simulink model "URM_IOKU_3b"  (R2014a)
settings: Solver=ode45  StartTime=0.0  StopTime=18  RelTol=1e-3
values from neighbouring files (symbols this model uses):
  a1 = 2    [URM_SP.m]
  a2 = 1.5    [URM_SP.m]
  a3 = 0.5    [URM_SP.m]
  D = linspace(d1,d2,n)    [URM_SP.m]
libraries: mblibv1 x12, simulink x3
settings Model: Creator=kajak_000  LastModifiedBy=kajak_000
settings SimMechanicsCC: VisDuringSimulation=on

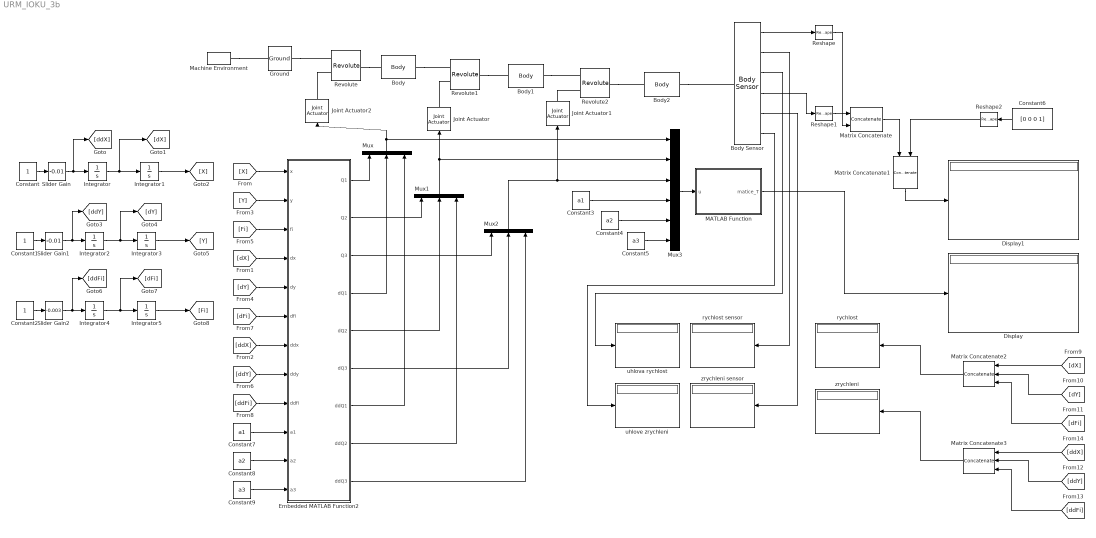
== system URM_IOKU_3b ==
  Body : mblibv1/Bodies/Body  LConnTagsString=CS1  RConnTagsString=CS2  UpdateFromCAD=off  DialogClass=MechanicalBodyBlock  Mass=1  MassUnits=kg  InertiaUnits=kg*m^2  Inertia=eye(3)  Shape=Cylinder  ShapeDims=[1 1]  ShapeUnits=m  ShapeUse=false  Density=1  DensityUnits=kg/m^3  DensityUse=false  GraphicsMode=MACHINE_DEFAULT  BodyColorSelMode=MACHINE_DEFAULT  BodyColor=[1 0 0]  AttachedToCS=CG  CG=Left$CG$rameno1.CG$WORLD$WORLD$m$[0 0 0]$Euler X-Y-Z$deg$WORLD$false$none  WorkingFrames=Left$CS1$rameno1.A$World$World$m$[0 0 0]$Euler X-Y-Z$deg$WORLD$true$none#Right$CS2$rameno1.B$World$World$m$[0 0 0]$Euler X-Y-Z$deg$WORLD$true$none  CGPos=rameno1.CG  CGRot=[0 0 0]  CS0Pos=[]  CS0Rot=[]  CS1Pos=rameno1.A  CS1Rot=[0 0 0]  CS2Pos=rameno1.B  CS2Rot=[0 0 0]  CS3Pos=[]  CS3Rot=[]  CS4Pos=[]  CS4Rot=[]  CS5Pos=[]  CS5Rot=[]  CS6Pos=[]  CS6Rot=[]  CS7Pos=[]  CS7Rot=[]  CS8Pos=[]  CS8Rot=[]  CS9Pos=[]  CS9Rot=[]  CS10Pos=[]  CS10Rot=[]  CS11Pos=[]  CS11Rot=[]  CS12Pos=[]  CS12Rot=[]  CS13Pos=[]  CS13Rot=[]  CS14Pos=[]  CS14Rot=[]  CS15Pos=[]  CS15Rot=[]  CS16Pos=[]  CS16Rot=[]  CS17Pos=[]  CS17Rot=[]  CS18Pos=[]  CS18Rot=[]  CS19Pos=[]  CS19Rot=[]  CS20Pos=[]  CS20Rot=[]
  Body Sensor : mblibv1/Sensors &  Actuators/Body Sensor  UpdateFromCAD=off  PhysicalDomain=Mechanical  PortType=blob  Muxed=off  Pose=on  Angle=on  AngleUnits=deg  ArcVelocity=on  ArcVelocityUnits=rad/s  ArcAcceleration=on  ArcAccelerationUnits=rad/s^2  CoordPosition=on  CoordPositionUnits=m  Velocity=on  VelocityUnits=m/s  Acceleration=on  AccelerationUnits=m/s^2  Quaternion=on  QuaternionDT=off  QuaternionDDT=off  QuaternionUnits=off  OutputVector="[ 3  3  3  9  3  3]"  ActiveIO=on  Width=24  DialogClass=MechanicalSensorBlock  ReferenceFrame=Absolute (World)
  Body1 : mblibv1/Bodies/Body  LConnTagsString=CS1  RConnTagsString=CS2  UpdateFromCAD=off  DialogClass=MechanicalBodyBlock  Mass=1  MassUnits=kg  InertiaUnits=kg*m^2  Inertia=eye(3)  Shape=Cylinder  ShapeDims=[1 1]  ShapeUnits=m  ShapeUse=false  Density=1  DensityUnits=kg/m^3  DensityUse=false  GraphicsMode=MACHINE_DEFAULT  BodyColorSelMode=MACHINE_DEFAULT  BodyColor=[1 0 0]  AttachedToCS=CG  CG=Left$CG$rameno2.CG$WORLD$WORLD$m$[0 0 0]$Euler X-Y-Z$deg$WORLD$false$none  WorkingFrames=Left$CS1$rameno2.A$World$World$m$[0 0 0]$Euler X-Y-Z$deg$WORLD$true$none#Right$CS2$rameno2.B$World$World$m$[0 0 0]$Euler X-Y-Z$deg$WORLD$true$none  CGPos=rameno2.CG  CGRot=[0 0 0]  CS0Pos=[]  CS0Rot=[]  CS1Pos=rameno2.A  CS1Rot=[0 0 0]  CS2Pos=rameno2.B  CS2Rot=[0 0 0]  CS3Pos=[]  CS3Rot=[]  CS4Pos=[]  CS4Rot=[]  CS5Pos=[]  CS5Rot=[]  CS6Pos=[]  CS6Rot=[]  CS7Pos=[]  CS7Rot=[]  CS8Pos=[]  CS8Rot=[]  CS9Pos=[]  CS9Rot=[]  CS10Pos=[]  CS10Rot=[]  CS11Pos=[]  CS11Rot=[]  CS12Pos=[]  CS12Rot=[]  CS13Pos=[]  CS13Rot=[]  CS14Pos=[]  CS14Rot=[]  CS15Pos=[]  CS15Rot=[]  CS16Pos=[]  CS16Rot=[]  CS17Pos=[]  CS17Rot=[]  CS18Pos=[]  CS18Rot=[]  CS19Pos=[]  CS19Rot=[]  CS20Pos=[]  CS20Rot=[]
  Body2 : mblibv1/Bodies/Body  LConnTagsString=CS1  RConnTagsString=CS2  UpdateFromCAD=off  DialogClass=MechanicalBodyBlock  Mass=1  MassUnits=kg  InertiaUnits=kg*m^2  Inertia=eye(3)  Shape=Cylinder  ShapeDims=[1 1]  ShapeUnits=m  ShapeUse=false  Density=1  DensityUnits=kg/m^3  DensityUse=false  GraphicsMode=MACHINE_DEFAULT  BodyColorSelMode=MACHINE_DEFAULT  BodyColor=[1 0 0]  AttachedToCS=CG  CG=Left$CG$rameno3.CG$WORLD$WORLD$m$[0 0 0]$Euler X-Y-Z$deg$WORLD$false$none  WorkingFrames=Left$CS1$rameno3.A$World$World$m$[0 0 0]$Euler X-Y-Z$deg$WORLD$true$none#Right$CS2$rameno3.B$World$World$m$[0 0 0]$Euler X-Y-Z$deg$WORLD$true$none  CGPos=rameno3.CG  CGRot=[0 0 0]  CS0Pos=[]  CS0Rot=[]  CS1Pos=rameno3.A  CS1Rot=[0 0 0]  CS2Pos=rameno3.B  CS2Rot=[0 0 0]  CS3Pos=[]  CS3Rot=[]  CS4Pos=[]  CS4Rot=[]  CS5Pos=[]  CS5Rot=[]  CS6Pos=[]  CS6Rot=[]  CS7Pos=[]  CS7Rot=[]  CS8Pos=[]  CS8Rot=[]  CS9Pos=[]  CS9Rot=[]  CS10Pos=[]  CS10Rot=[]  CS11Pos=[]  CS11Rot=[]  CS12Pos=[]  CS12Rot=[]  CS13Pos=[]  CS13Rot=[]  CS14Pos=[]  CS14Rot=[]  CS15Pos=[]  CS15Rot=[]  CS16Pos=[]  CS16Rot=[]  CS17Pos=[]  CS17Rot=[]  CS18Pos=[]  CS18Rot=[]  CS19Pos=[]  CS19Rot=[]  CS20Pos=[]  CS20Rot=[]
  Constant : Constant
  Constant1 : Constant
  Constant2 : Constant
  Constant3 : Constant  Value=a1
  Constant4 : Constant  Value=a2
  Constant5 : Constant  Value=a3
  Constant6 : Constant  Value=[0 0 0 1]
  Constant7 : Constant  Value=a1
  Constant8 : Constant  Value=a2
  Constant9 : Constant  Value=a3
  Display : Display
  Display1 : Display
  Embedded MATLAB Function2 : MATLAB Function  TreatAsAtomicUnit=on
  Ground : mblibv1/Bodies/Ground  UpdateFromCAD=off  LeftPortType=env  RightPortType=workingframe  PhysicalDomain=Mechanical  DialogClass=GroundBlock  CoordPosition=rameno1.A  CoordPositionUnits=m  StateVectorMgrId=7  MachineId=[8 0]  ShowEnvPort=on  ParameterChecksum=[1572609533, 1849027617, 4062556937, 1555680548]  TopologyChecksum=[1622869580, 615649969, 3102652873, 2552126148]
  Integrator{,1..5} (6 alike) : Integrator
  Joint Actuator : mblibv1/Sensors &  Actuators/Joint Actuator  UpdateFromCAD=off  PhysicalDomain=Mechanical  PortType=blob  ActuationStyle=Motion  AngleUnits=rad  ArcVelocityUnits=rad/s  ArcAccelerationUnits=rad/s^2  CoordPositionUnits=m  VelocityUnits=m/s  AccelerationUnits=m/s^2  ForceUnits=N  TorqueUnits=N*m  ActiveIO=on  Width=3  DialogClass=MechanicalActuatorBlock  Primitive=R1  ReferenceFrame=Absolute (World)
  Joint Actuator1 : mblibv1/Sensors &  Actuators/Joint Actuator  UpdateFromCAD=off  PhysicalDomain=Mechanical  PortType=blob  ActuationStyle=Motion  AngleUnits=rad  ArcVelocityUnits=rad/s  ArcAccelerationUnits=rad/s^2  CoordPositionUnits=m  VelocityUnits=m/s  AccelerationUnits=m/s^2  ForceUnits=N  TorqueUnits=N*m  ActiveIO=on  Width=3  DialogClass=MechanicalActuatorBlock  Primitive=R1  ReferenceFrame=Absolute (World)
  Joint Actuator2 : mblibv1/Sensors &  Actuators/Joint Actuator  UpdateFromCAD=off  PhysicalDomain=Mechanical  PortType=blob  ActuationStyle=Motion  AngleUnits=rad  ArcVelocityUnits=rad/s  ArcAccelerationUnits=rad/s^2  CoordPositionUnits=m  VelocityUnits=m/s  AccelerationUnits=m/s^2  ForceUnits=N  TorqueUnits=N*m  ActiveIO=on  Width=3  DialogClass=MechanicalActuatorBlock  Primitive=R1  ReferenceFrame=Absolute (World)
  MATLAB Function : MATLAB Function  TreatAsAtomicUnit=on
  Machine Environment : mblibv1/Bodies/Machine Environment  PortType=env  PhysicalDomain=Mechanical  DialogTemplateClass=MECH.MachineEnvironment  SyncWhenCopied=off  Gravity=[0 0 0]  GravityUnits=m/s^2  GravityAsSignal=off  Dimensionality=Auto-detect  AnalysisType=Forward dynamics  LinearAssemblyTolerance=1e-3  LinearAssemblyToleranceUnits=m  AngularAssemblyTolerance=1e-3  AngularAssemblyToleranceUnits=rad  ConstraintSolverType=Stabilizing  ConstraintRelTolerance=1e-4  ConstraintAbsTolerance=1e-4  UseRobustSingularityHandling=off  RedundancyAnalysisToleranceType=Automatically select tolerance  RedundancyAnalysisTolerance=1e-14  StatePerturbationType=Fixed  PerturbationSize=1e-5  VisualizeMachine=on  BodyVisualizationType=Use model default body geometries  BodyColorSelMode=Use model default  DefaultBodyColor=[1 0 0]
  Matrix Concatenate : Concatenate  Mode=Multidimensional array  ConcatenateDimension=2
  Matrix Concatenate1 : Concatenate  Mode=Multidimensional array
  Matrix Concatenate2 : Concatenate  NumInputs=3  ConcatenateDimension=2
  Matrix Concatenate3 : Concatenate  NumInputs=3  ConcatenateDimension=2
  Mux : Mux  Inputs=3
  Mux1 : Mux  Inputs=3
  Mux2 : Mux  Inputs=3
  Mux3 : Mux  Inputs=6
  Reshape : Reshape  OutputDimensionality=Column vector (2-D)
  Reshape1 : Reshape  OutputDimensionality=Customize  OutputDimensions=[3,3]
  Reshape2 : Reshape  OutputDimensionality=Row vector (2-D)  OutputDimensions=[3,1]
  Revolute : mblibv1/Joints/Revolute  LConnTagsString=__newl0|SA1  RConnTagsString=__newr0  UpdateFromCAD=off  NumSAPorts=1  CutJoint=off  MarkAsCut=off  Primitives=prismatic  PrimitiveProps=R1$World$rameno1.osa$revolute  DialogClass=JointBlock  R1Axis=rameno1.osa
  Revolute1 : mblibv1/Joints/Revolute  LConnTagsString=__newl0|SA1  RConnTagsString=__newr0  UpdateFromCAD=off  NumSAPorts=1  CutJoint=off  MarkAsCut=off  Primitives=prismatic  PrimitiveProps=R1$World$rameno2.osa$revolute  DialogClass=JointBlock  R1Axis=rameno2.osa
  Revolute2 : mblibv1/Joints/Revolute  LConnTagsString=__newl0|SA1  RConnTagsString=__newr0  UpdateFromCAD=off  NumSAPorts=1  CutJoint=off  MarkAsCut=off  Primitives=prismatic  PrimitiveProps=R1$World$rameno3.osa$revolute  DialogClass=JointBlock  R1Axis=rameno3.osa
  Slider Gain : simulink/Math Operations/Slider Gain  low=-2  gain=-0.01  high=2
  Slider Gain1 : simulink/Math Operations/Slider Gain  low=-2  gain=-0.01  high=2
  Slider Gain2 : simulink/Math Operations/Slider Gain  low=-2  gain=-0.003  high=2
  rychlost : Display
  rychlost sensor : Display
  uhlova rychlost : Display
  uhlove zrychleni : Display
  zrychleni : Display
  zrychleni sensor : Display
  wires:
  Slider Gain/1 -> [ddX], Integrator/1
  Constant/1 -> Slider Gain/1
  Constant3/1 -> Mux3/4
  Constant4/1 -> Mux3/5
  Constant5/1 -> Mux3/6
  Mux3/1 -> MATLAB Function/1(u)
  MATLAB Function/1(matice_T) -> Display/1
  Body Sensor/1 -> Reshape/1
  Body Sensor/4 -> Reshape1/1
  Reshape1/1 -> Matrix Concatenate/1
  Reshape/1 -> Matrix Concatenate/2
  Constant6/1 -> Reshape2/1
  Matrix Concatenate/1 -> Matrix Concatenate1/1
  Reshape2/1 -> Matrix Concatenate1/2
  Matrix Concatenate1/1 -> Display1/1
  Integrator/1 -> [dX], Integrator1/1
  Slider Gain1/1 -> [ddY], Integrator2/1
  Constant1/1 -> Slider Gain1/1
  Integrator2/1 -> [dY], Integrator3/1
  Body Sensor/2 -> rychlost sensor/1
  Body Sensor/5 -> zrychleni sensor/1
  Body Sensor/3 -> uhlova rychlost/1
  Body Sensor/6 -> uhlove zrychleni/1
  [X] -> Embedded MATLAB Function2/1(x)
  Integrator1/1 -> [X]
  Integrator3/1 -> [Y]
  Slider Gain2/1 -> [ddFi], Integrator4/1
  Constant2/1 -> Slider Gain2/1
  Integrator4/1 -> [dFi], Integrator5/1
  Integrator5/1 -> [Fi]
  Mux/1 -> Joint Actuator2/1, Mux3/1
  Mux1/1 -> Joint Actuator/1, Mux3/2
  Mux2/1 -> Joint Actuator1/1, Mux3/3
  Matrix Concatenate2/1 -> rychlost/1
  [dX] -> Matrix Concatenate2/1
  [dY] -> Matrix Concatenate2/2
  [dFi] -> Matrix Concatenate2/3
  Matrix Concatenate3/1 -> zrychleni/1
  [ddX] -> Matrix Concatenate3/1
  [ddY] -> Matrix Concatenate3/2
  [ddFi] -> Matrix Concatenate3/3
  [Y] -> Embedded MATLAB Function2/2(y)
  [dX] -> Embedded MATLAB Function2/4(dx)
  [dY] -> Embedded MATLAB Function2/5(dy)
  [dFi] -> Embedded MATLAB Function2/6(dfi)
  [ddY] -> Embedded MATLAB Function2/8(ddy)
  [ddX] -> Embedded MATLAB Function2/7(ddx)
  [Fi] -> Embedded MATLAB Function2/3(fi)
  [ddFi] -> Embedded MATLAB Function2/9(ddfi)
  Constant7/1 -> Embedded MATLAB Function2/10(a1)
  Constant8/1 -> Embedded MATLAB Function2/11(a2)
  Constant9/1 -> Embedded MATLAB Function2/12(a3)
  Embedded MATLAB Function2/1(Q1) -> Mux/1
  Embedded MATLAB Function2/4(dQ1) -> Mux/2
  Embedded MATLAB Function2/7(ddQ1) -> Mux/3
  Embedded MATLAB Function2/2(Q2) -> Mux1/1
  Embedded MATLAB Function2/5(dQ2) -> Mux1/2
  Embedded MATLAB Function2/8(ddQ2) -> Mux1/3
  Embedded MATLAB Function2/3(Q3) -> Mux2/1
  Embedded MATLAB Function2/6(dQ3) -> Mux2/2
  Embedded MATLAB Function2/9(ddQ3) -> Mux2/3
  connections:
  Machine Environment/RConn1 -- Ground/LConn1
  Ground/RConn1 -- Revolute/LConn1
  Revolute/RConn1 -- Body/LConn1
  Body/RConn1 -- Revolute1/LConn1
  Revolute1/RConn1 -- Body1/LConn1
  Body1/RConn1 -- Revolute2/LConn1
  Revolute2/RConn1 -- Body2/LConn1
  Body2/RConn1 -- Body Sensor/LConn1
  Joint Actuator/RConn1 -- Revolute1/LConn2
  Joint Actuator1/RConn1 -- Revolute2/LConn2
  Joint Actuator2/RConn1 -- Revolute/LConn2

== matlab function URM_IOKU_3b/MATLAB Function ==
  data: u input; matice_T output
function matice_T = DGM_funkce(u)
Q1 = u(1); % poloha
Q2 = u(4);
Q3 = u(7);
a1 = u(10);
a2 = u(11);
a3 = u(12);
matice_T = zeros(4);

x = a3 * cos(Q1 + Q2 + Q3) + a2 * cos(Q1 + Q2) + a1 * cos(Q1);
y = a3 * sin(Q1 + Q2 + Q3) + a2 * sin(Q1 + Q2) + a1 * sin(Q1);
vysledny_uhel = Q1 + Q2 + Q3; 

matice_T = [ cos(vysledny_uhel),-sin(vysledny_uhel),0,x;
            sin(vysledny_uhel),cos(vysledny_uhel),0,y;
            0,0,1,0;
            0,0,0,1 ];
       
end

== matlab function URM_IOKU_3b/Embedded MATLAB Function2 ==
  data: Q1 output; Q2 output; Q3 output; dQ1 output; dQ2 output; dQ3 output; ddQ1 output; ddQ2 output; ddQ3 output; x input; y input; fi input; dx input; dy input; dfi input; ddx input; ddy input; ddfi input; a1 input; a2 input; a3 input
function [Q1, Q2, Q3, dQ1, dQ2, dQ3, ddQ1, ddQ2, ddQ3] = IOKU(x, y, fi, dx, dy, dfi, ddx, ddy, ddfi, a1, a2, a3)
% vypocet Q2
cosQ2 = ((x - a3*cos(fi))^2 + (y - a3*sin(fi))^2 - a1^2 - a2^2)/(2 * a1 * a2);
sinQ2 = -(sqrt((1 - cosQ2^2)));
Q2 = atan2(sinQ2, cosQ2);

% vypocet Q1
A = [-a2 * sinQ2, a2 * cosQ2 + a1; a2 * cosQ2 + a1, a2 * sinQ2];
B = [x - a3*cos(fi); y - a3*sin(fi)];
V = A^(-1) * B;
Q1 = atan2(V(1), V(2));

% vypocet Q3
Q3 = fi - Q1 - Q2;
% rychlost dX
jQ = [-a3 * sin(Q1 + Q2 + Q3) - a2 * sin(Q1 + Q2) - a1 * sin(Q1), -a3 * sin(Q1 + Q2 + Q3) - a2 * sin(Q1 + Q2), -a3 * sin(Q1 + Q2 + Q3);...
    a3 * cos(Q1 + Q2 + Q3) + a2 * cos(Q1 + Q2) + a1 * cos(Q1), a3 * cos(Q1 + Q2 + Q3) + a2 * cos(Q1 + Q2), a3 * cos(Q1 + Q2 + Q3);...
    1, 1, 1];
dX = [dx; dy; dfi];
dQ = jQ^(-1) * dX;
dQ1 = dQ(1);
dQ2 = dQ(2);
dQ3 = dQ(3);

% zrychleni ddX
djQ = [-a3*cos(Q1+Q2+Q3)*(dQ1+dQ2+dQ3) - a2*cos(Q1+Q2)*(dQ1+dQ2) - a1*cos(Q1)*dQ1, -a3*cos(Q1+Q2+Q3)*(dQ1+dQ2+dQ3) - a2*cos(Q1+Q2)*(dQ1+dQ2), -a3*cos(Q1+Q2+Q3)*(dQ1+dQ2+dQ3);...
    -a3*sin(Q1+Q2+Q3)*(dQ1+dQ2+dQ3) - a2*sin(Q1+Q2)*(dQ1+dQ2) - a1*sin(Q1)*dQ1, -a3*sin(Q1+Q2+Q3)*(dQ1+dQ2+dQ3) - a2*sin(Q1+Q2)*(dQ1+dQ2), -a3*sin(Q1+Q2+Q3)*(dQ1+dQ2+dQ3);...
    0, 0, 0];
ddX = [ddx; ddy; ddfi];
ddQ = jQ^(-1) * (ddX - djQ * dQ);
ddQ1 = ddQ(1);
ddQ2 = ddQ(2);
ddQ3 = ddQ(3);
end
